simulink model "full_system"  (R2022b)
settings: Solver=FixedStepAuto  StartTime=0.0  StopTime=10.0  FixedStep=0.001  RelTol=1e-4
values from neighbouring files (symbols this model uses):
  initial_conditions_1 = [8, 8, 0]    [init.m]
  initial_conditions_2 = [6, 3, 2*pi]    [init.m]
  initial_conditions_3 = [-8, -8, 3*pi/2]    [init.m]
undefined symbols (not defined in the file or in its folder): distance_threshold
settings Model: Creator=gotta  LastModifiedBy=Edp

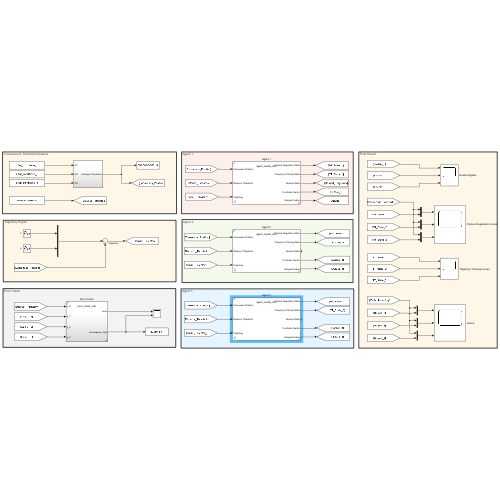
[thumbnail: Simulink's stored preview of the top-level diagram]
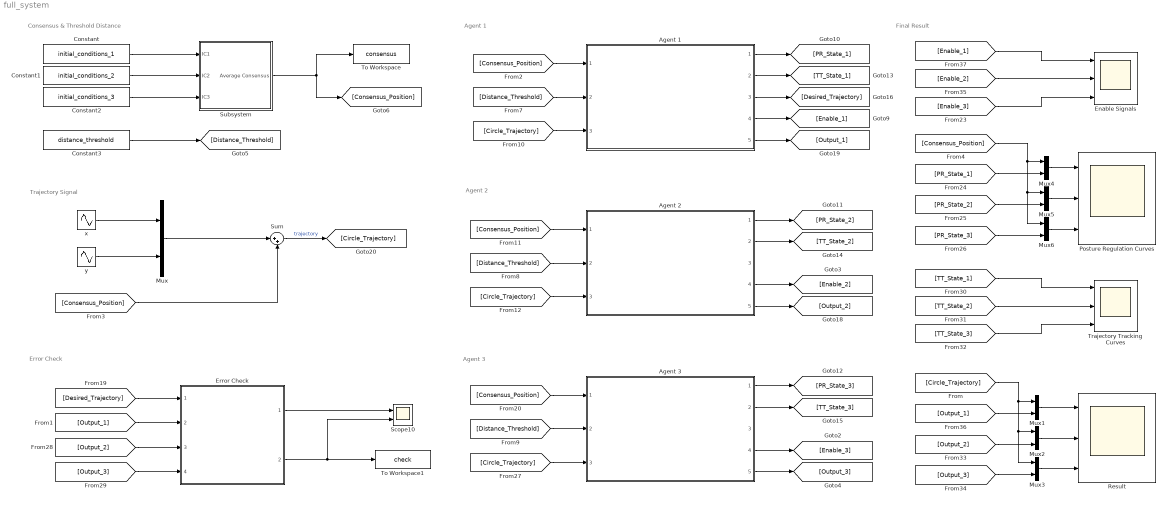
== system full_system ==
  note: Trajectory Signal
  note: Error Check
  note: Agent 3
  note: Agent 2
  note: Agent 1
  note: Consensus & Threshold Distance
  note: Final Result
  Agent 1 : Subsystem  ReferencedSubsystem=agent_model_sub  InitialCondition_trans=initial_conditions_trans_1  InitialCondition=initial_conditions_1
  Agent 2 : Subsystem  ReferencedSubsystem=agent_model_sub  InitialCondition_trans=initial_conditions_trans_2  InitialCondition=initial_conditions_2
  Agent 3 : Subsystem  ReferencedSubsystem=agent_model_sub  InitialCondition_trans=initial_conditions_trans_3  InitialCondition=initial_conditions_3
  Constant : Constant  Value=initial_conditions_1
  Constant1 : Constant  Value=initial_conditions_2
  Constant2 : Constant  Value=initial_conditions_3
  Constant3 : Constant  Value=distance_threshold
  Enable Signals : Scope  NumInputPorts=3
  Error Check : Subsystem  ReferencedSubsystem=error_check_sub
  Mux{,1..6} (7 alike) : Mux  Inputs=2
  Posture Regulation Curves : Scope  NumInputPorts=3
  Result : Scope  NumInputPorts=3
  Scope10 : Scope  NumInputPorts=2
  Subsystem : Subsystem
  Sum : Sum  Inputs=|++
  To Workspace : ToWorkspace  VariableName=consensus  SaveFormat=Structure With Time  SampleTime=-1
  To Workspace1 : ToWorkspace  VariableName=check  SaveFormat=Structure With Time  SampleTime=-1
  Trajectory Tracking Curves : Scope  NumInputPorts=3
  x : Sin  SampleTime=0
  y : Sin  Phase=pi/2  SampleTime=0
  wires:
  Constant1/1 -> Subsystem/2(IC2)
  Constant/1 -> Subsystem/1(IC1)
  Constant2/1 -> Subsystem/3(IC3)
  Constant3/1 -> [Distance_Threshold]
  Agent 1/4 -> [Enable_1]
  Agent 1/1 -> [PR_State_1]
  [Distance_Threshold] -> Agent 1/2
  Agent 1/2 -> [TT_State_1]
  [Consensus_Position] -> Agent 2/1
  Agent 2/2 -> [TT_State_2]
  [Distance_Threshold] -> Agent 2/2
  Agent 2/4 -> [Enable_2]
  Agent 2/1 -> [PR_State_2]
  Agent 3/2 -> [TT_State_3]
  Agent 3/1 -> [PR_State_3]
  [Distance_Threshold] -> Agent 3/2
  Agent 3/4 -> [Enable_3]
  [Desired_Trajectory] -> Error Check/1
  Error Check/2 -> Scope10/2, To Workspace1/1
  Error Check/1 -> Scope10/1
  Agent 1/3 -> [Desired_Trajectory]
  Agent 1/5 -> [Output_1]
  Agent 2/5 -> [Output_2]
  Agent 3/5 -> [Output_3]
  x/1 -> Mux/1
  y/1 -> Mux/2
  [Consensus_Position] -> Agent 1/1
  Sum/1 -> [Circle_Trajectory]  "trajectory"
  [Circle_Trajectory] -> Agent 1/3
  [Circle_Trajectory] -> Agent 2/3
  [Consensus_Position] -> Agent 3/1
  [Circle_Trajectory] -> Agent 3/3
  Mux/1 -> Sum/1
  [Consensus_Position] -> Sum/2
  [Output_3] -> Error Check/4
  [Output_2] -> Error Check/3
  [Output_1] -> Error Check/2
  [Enable_2] -> Enable Signals/2
  [Enable_1] -> Enable Signals/1
  [Enable_3] -> Enable Signals/3
  [TT_State_3] -> Trajectory Tracking Curves/3
  [TT_State_2] -> Trajectory Tracking Curves/2
  [TT_State_1] -> Trajectory Tracking Curves/1
  Mux1/1 -> Result/1
  [Output_1] -> Mux1/2
  [Circle_Trajectory] -> Mux2/1, Mux3/1, Mux1/1
  Mux3/1 -> Result/3
  Mux2/1 -> Result/2
  [Output_2] -> Mux2/2
  [Output_3] -> Mux3/2
  [PR_State_1] -> Mux4/2
  Mux6/1 -> Posture Regulation Curves/3
  Mux5/1 -> Posture Regulation Curves/2
  [Consensus_Position] -> Mux5/1, Mux6/1, Mux4/1
  [PR_State_2] -> Mux5/2
  [PR_State_3] -> Mux6/2
  Mux4/1 -> Posture Regulation Curves/1
  Subsystem/1(Average Consensus) -> [Consensus_Position], To Workspace/1

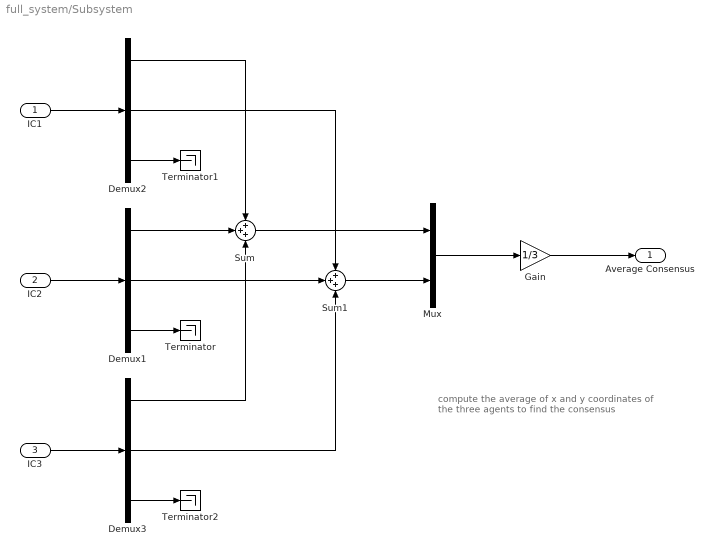
== system full_system/Subsystem ==
  note: compute the average of x and y coordinates
      | of the three agents to find the consensus
  IC1 : Inport
  IC2 : Inport  Port=2
  IC3 : Inport  Port=3
  Demux1 : Demux  Outputs=3
  Demux2 : Demux  Outputs=3
  Demux3 : Demux  Outputs=3
  Gain : Gain  Gain=1/3
  Mux : Mux  Inputs=2
  Sum : Sum  Inputs=+++
  Sum1 : Sum  Inputs=+++
  Terminator : Terminator
  Terminator1 : Terminator
  Terminator2 : Terminator
  Average Consensus : Outport
  wires:
  IC2/1 -> Demux1/1
  Demux1/1 -> Sum/2
  Demux1/2 -> Sum1/2
  Demux1/3 -> Terminator/1
  IC1/1 -> Demux2/1
  Demux2/1 -> Sum/1
  Demux2/2 -> Sum1/1
  Demux2/3 -> Terminator1/1
  Mux/1 -> Gain/1
  Sum/1 -> Mux/1
  Sum1/1 -> Mux/2
  Demux3/3 -> Terminator2/1
  Demux3/2 -> Sum1/3
  Demux3/1 -> Sum/3
  IC3/1 -> Demux3/1
  Gain/1 -> Average Consensus/1
